simulink model "FB_checkout"  (Simulink 9.2)
settings: Solver=FixedStepDiscrete  StartTime=0.0  StopTime=10  FixedStep=SIM_dt  RelTol=1e-3
values from neighbouring files (symbols this model uses):
  SIM_dt = 0.01    [init_secOrdFilt_checkout.m]    (also in init_secOrdSS_checkout.m = 0.001)
undefined symbols (not defined in the file or in its folder): FB_kd, FB_ki, FB_kp
libraries: simulink x1
settings Model: Creator=coewal  LastModifiedBy=coewal
settings DataIOCC: LimitDataPoints=off  SaveFormat=Dataset  SignalLoggingSaveFormat=Dataset
settings OptimizationCC: LifeSpan=auto
settings DebuggingCC: UnderspecifiedInitializationDetection=Simplified  MergeDetectMultiDrivingBlocksExec=error  FcnCallInpInsideContextMsg=error  StateNameClashWarn=none  SFUnexpectedBacktrackingDiag=error  SFNoUnconditionalDefaultTransitionDiag=error  SFExecutionAtInitializationDiag=warning
settings HardwareCC: ProdBitPerPointer=64  ProdBitPerSizeT=64  ProdBitPerPtrDiffT=64  ProdLargestAtomicFloat=Float  ProdIntDivRoundTo=Zero  ProdEndianess=LittleEndian  ProdWordSize=64  ProdHWDeviceType=Intel->x86-64 (Windows64)
settings ModelReferenceCC: PropagateSignalLabelsOutOfModel=on
settings SFSimCC: SimUseLocalCustomCode=on
settings RTWCC: RTWUseLocalCustomCode=on
settings CodeAppCC: StateflowObjectComments=off
settings GRTTargetCC: TargetLangStandard=C99 (ISO)  GeneratePreprocessorConditionals=Use local settings  CombineOutputUpdateFcns=on  GRTInterface=off
settings ConfigComp: CovMetricSettings=dwe  CovHtmlReporting=off  CovSaveCumulativeToWorkspaceVar=off  CovSaveSingleToWorkspaceVar=off  CovExternalEMLEnable=on

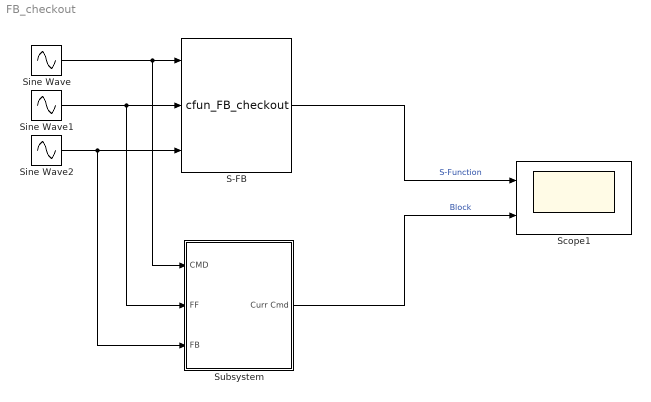
== system FB_checkout ==
  S-FB : S-Function  FunctionName=cfun_FB_checkout  Parameters=SIM_dt, FB_kp, FB_ki, FB_kd  SFunctionModules='FB'  SFunctionDeploymentMode=off  EnableBusSupport=off
  Scope1 : Scope  NumInputPorts=2
  Sine Wave : Sin  Amplitude=pi/180  Frequency=5  SampleTime=SIM_dt
  Sine Wave1 : Sin  Amplitude=pi/180  Frequency=2  Phase=1  SampleTime=SIM_dt
  Sine Wave2 : Sin  Amplitude=pi/180  Frequency=10  Phase=-1  SampleTime=SIM_dt
  Subsystem : Subsystem
  wires:
  Sine Wave/1 -> Subsystem/1(CMD), S-FB/1
  Sine Wave1/1 -> Subsystem/2(FF), S-FB/2
  Sine Wave2/1 -> Subsystem/3(FB), S-FB/3
  S-FB/1 -> Scope1/1  "S-Function"
  Subsystem/1(Curr Cmd) -> Scope1/2  "Block"

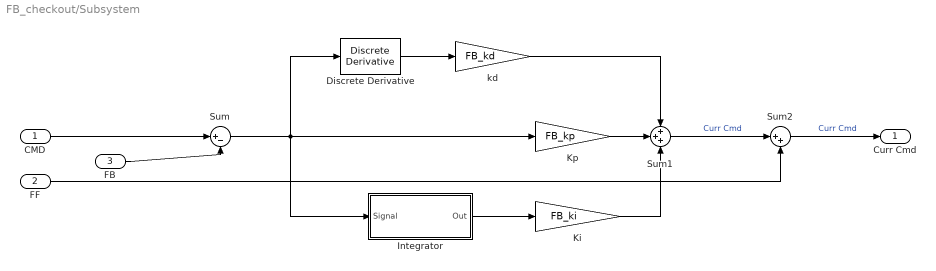
== system FB_checkout/Subsystem ==
  CMD : Inport
  FF : Inport  Port=2
  FB : Inport  Port=3
  Discrete Derivative : simulink/Discrete/Discrete Derivative  gainval=1.0  ICPrevScaledInput=0.0  OutMin=[]  OutMax=[]  OutDataType=fixdt(1, 16)  OutScaling=2^-10  DoSatur=off
  Integrator : Subsystem
  Ki : Gain  Gain=FB_ki
  Kp : Gain  Gain=FB_kp
  Sum : Sum  Inputs=|+-
  Sum1 : Sum  Inputs=+++
  Sum2 : Sum  Inputs=|++
  kd : Gain  Gain=FB_kd
  Curr Cmd : Outport
  wires:
  Kp/1 -> Sum1/2
  Discrete Derivative/1 -> kd/1
  Integrator/1(Out) -> Ki/1
  Sum/1 -> Discrete Derivative/1, Integrator/1(Signal), Kp/1
  Sum2/1 -> Curr Cmd/1  "Curr Cmd"
  FB/1 -> Sum/2
  kd/1 -> Sum1/1
  Sum1/1 -> Sum2/1  "Curr Cmd"
  FF/1 -> Sum2/2
  Ki/1 -> Sum1/3
  CMD/1 -> Sum/1

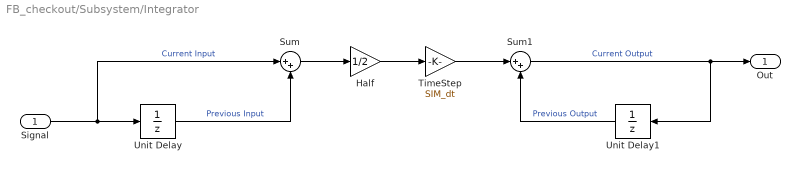
== system FB_checkout/Subsystem/Integrator ==
  Signal : Inport
  Half : Gain  Gain=1/2
  Sum : Sum  Inputs=|++
  Sum1 : Sum  Inputs=|++
  TimeStep : Gain  Gain=SIM_dt
  Unit Delay : UnitDelay  SampleTime=-1
  Unit Delay1 : UnitDelay  SampleTime=-1
  Out : Outport
  wires:
  Signal/1 -> Sum/1, Unit Delay/1  "Current Input"
  Unit Delay/1 -> Sum/2  "Previous Input"
  Sum/1 -> Half/1
  Half/1 -> TimeStep/1
  TimeStep/1 -> Sum1/1
  Sum1/1 -> Unit Delay1/1, Out/1  "Current Output"
  Unit Delay1/1 -> Sum1/2  "Previous Output"
